simulink library "AssistOn_Gait_Lib"  (R2020a)
settings: Solver=VariableStepAuto  StartTime=0.0  StopTime=10.0  RelTol=1e-3
libraries: xpcethercatlib x12, simulink x3, slrtlib x1
settings Model: Creator=AliYasar  LastModifiedBy=AliYasar

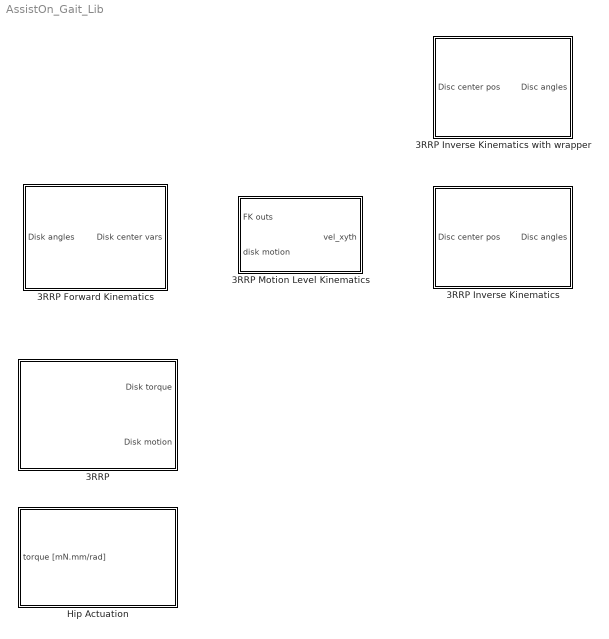
== system AssistOn_Gait_Lib ==
  3RRP : Subsystem  TreatAsAtomicUnit=on
  3RRP Forward Kinematics : Subsystem
      settings: MinAlgLoopOccurrences=on
  3RRP Inverse Kinematics : Subsystem
      settings: MinAlgLoopOccurrences=on
  3RRP Inverse Kinematics with wrapper : Subsystem
      settings: MinAlgLoopOccurrences=on
  3RRP Motion Level Kinematics : Subsystem
  Hip Actuation : Subsystem

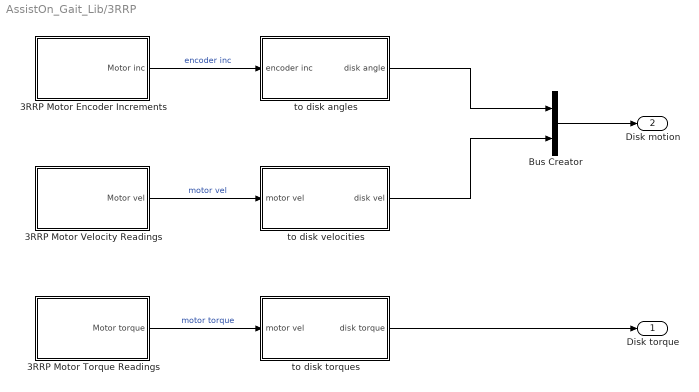
== system AssistOn_Gait_Lib/3RRP ==
  3RRP Motor Encoder Increments : Subsystem
  3RRP Motor Torque Readings : Subsystem
  3RRP Motor Velocity Readings : Subsystem
  Bus Creator : BusCreator  Inputs=2
  to disk angles : Subsystem
  to disk torques : Subsystem
  to disk velocities : Subsystem
  Disk torque : Outport  VectorParamsAs1DForOutWhenUnconnected=off
  Disk motion : Outport  Port=2  VectorParamsAs1DForOutWhenUnconnected=off
  wires:
  Bus Creator/1 -> Disk motion/1
  3RRP Motor Velocity Readings/1(Motor vel) -> to disk velocities/1(motor vel)  "motor vel"
  3RRP Motor Encoder Increments/1(Motor inc) -> to disk angles/1(encoder inc)  "encoder inc"
  to disk angles/1(disk angle) -> Bus Creator/1
  to disk velocities/1(disk vel) -> Bus Creator/2
  3RRP Motor Torque Readings/1(Motor torque) -> to disk torques/1(motor vel)  "motor torque"
  to disk torques/1(disk torque) -> Disk torque/1

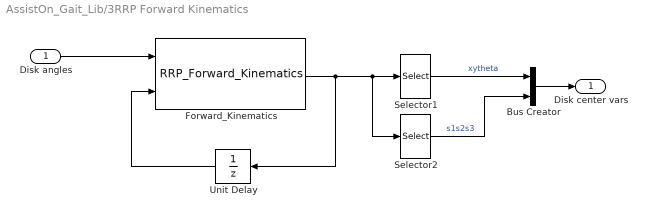
== system AssistOn_Gait_Lib/3RRP Forward Kinematics ==
  Disk angles : Inport
  Bus Creator : BusCreator  Inputs=2
  Forward_Kinematics : S-Function  FunctionName=RRP_Forward_Kinematics  SFunctionModules=RRP_Forward_Kinematics_wrapper  SFunctionDeploymentMode=off  EnableBusSupport=off
  Selector1 : Selector  InputPortWidth=6  IndexOptions=Index vector (dialog)  Indices=[1 2 3]  OutputSizes=1
  Selector2 : Selector  InputPortWidth=6  IndexOptions=Index vector (dialog)  Indices=[4 5 6]  OutputSizes=1
  Unit Delay : UnitDelay  InitialCondition=[0 0 0 151.28 151.28 151.28]  SampleTime=-1  HasFrameUpgradeWarning=on
  Disk center vars : Outport  VectorParamsAs1DForOutWhenUnconnected=off
  wires:
  Unit Delay/1 -> Forward_Kinematics/2
  Forward_Kinematics/1 -> Unit Delay/1, Selector2/1, Selector1/1
  Disk angles/1 -> Forward_Kinematics/1
  Bus Creator/1 -> Disk center vars/1
  Selector1/1 -> Bus Creator/1  "xytheta"
  Selector2/1 -> Bus Creator/2  "s1s2s3"

== system AssistOn_Gait_Lib/3RRP Inverse Kinematics ==
  Disc center pos : Inport
  S-Function : S-Function  FunctionName=RRP_Inverse_Kinematics  SFunctionModules='RRP_Inverse_Kinematics_wrapper'  SFunctionDeploymentMode=off  EnableBusSupport=off
  Unit Delay : UnitDelay  InitialCondition=[2*pi/3,-2*pi/3,0,151.28,151.28,151.28]  SampleTime=-1  HasFrameUpgradeWarning=on
  no op : Subsystem
  Disc angles : Outport
  wires:
  Disc center pos/1 -> S-Function/1
  Unit Delay/1 -> S-Function/2
  S-Function/1 -> no op/1(IK solution)
  no op/1(Pos) -> Disc angles/1
  no op/2(Corrected IK solution) -> Unit Delay/1

== system AssistOn_Gait_Lib/3RRP Inverse Kinematics with wrapper ==
  Disc center pos : Inport
  S-Function : S-Function  FunctionName=RRP_Inverse_Kinematics  SFunctionModules='RRP_Inverse_Kinematics_wrapper'  SFunctionDeploymentMode=off  EnableBusSupport=off
  Unit Delay : UnitDelay  InitialCondition=[2*pi/3,-2*pi/3,0,151.28,151.28,151.28]  SampleTime=-1  HasFrameUpgradeWarning=on
  "wrap position to [-pi, pi]" : Subsystem
  Disc angles : Outport
  wires:
  "wrap position to [-pi, pi]"/2(Corrected IK solution) -> Unit Delay/1
  "wrap position to [-pi, pi]"/1(Pos) -> Disc angles/1
  S-Function/1 -> "wrap position to [-pi, pi]"/1(IK solution)
  Unit Delay/1 -> S-Function/2
  Disc center pos/1 -> S-Function/1

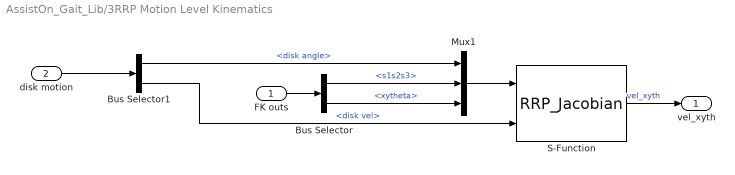
== system AssistOn_Gait_Lib/3RRP Motion Level Kinematics ==
  FK outs : Inport
  disk motion : Inport  Port=2
  Bus Selector : BusSelector  OutputSignals=s1s2s3,xytheta
  Bus Selector1 : BusSelector  OutputSignals=disk angle,disk vel
  Mux1 : Mux  Inputs=3
  S-Function : S-Function  FunctionName=RRP_Jacobian  SFunctionModules='RRP_Jacobian_wrapper'  SFunctionDeploymentMode=off  EnableBusSupport=off
  vel_xyth : Outport
  wires:
  Mux1/1 -> S-Function/1
  FK outs/1 -> Bus Selector/1
  S-Function/1 -> vel_xyth/1  "vel_xyth"
  disk motion/1 -> Bus Selector1/1
  Bus Selector/1 -> Mux1/2  "<s1s2s3>"
  Bus Selector/2 -> Mux1/3  "<xytheta>"
  Bus Selector1/1 -> Mux1/1  "<disk angle>"
  Bus Selector1/2 -> S-Function/2  "<disk vel>"

== system AssistOn_Gait_Lib/Hip Actuation ==
  torque [mN.mm/rad] : Inport
  M1 Target Torque : xpcethercatlib/EtherCAT PDO Transmit   Priority=3  sig_name=Drive 1 (MAXPOS).Module 1 (CST Mode).CST Outputs.Target Torque  sig_offset=656  sig_type=int16  type_size=16  sig_dim=1  device_id=0  sample_time=0.001000
      settings: SourceProductBaseCode=XP
  M2 Target Torque : xpcethercatlib/EtherCAT PDO Transmit   Priority=3  sig_name=Drive 2 (MAXPOS).Module 1 (CST Mode).CST Outputs.TargetTorque  sig_offset=768  sig_type=int16  type_size=16  sig_dim=1  device_id=0  sample_time=0.001000
      settings: SourceProductBaseCode=XP
  M3 Target Torque : xpcethercatlib/EtherCAT PDO Transmit   Priority=3  sig_name=Drive 3 (MAXPOS).Module 1 (CST Mode).CST Outputs.TargetTorque  sig_offset=880  sig_type=int16  type_size=16  sig_dim=1  device_id=0  sample_time=0.001000
      settings: SourceProductBaseCode=XP
  Target Torque : Subsystem
  wires:
  torque [mN.mm/rad]/1 -> Target Torque/1(torque)
  Target Torque/1(M1_torque) -> M1 Target Torque/1
  Target Torque/2(M2_torque) -> M2 Target Torque/1
  Target Torque/3(M3_torque) -> M3 Target Torque/1

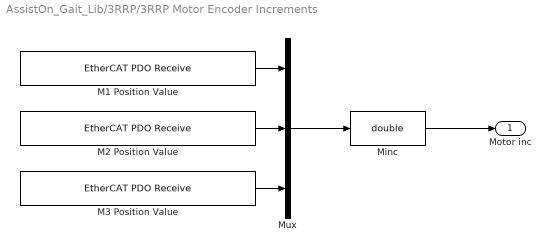
== system AssistOn_Gait_Lib/3RRP/3RRP Motor Encoder Increments ==
  M1 Position Value : xpcethercatlib/EtherCAT PDO Receive  Priority=2  sig_name=Drive 1 (MAXPOS).Module 1 (CST Mode).CST Inputs.PositionActualValue  sig_offset=568  sig_type=int32  type_size=32  sig_dim=1  device_id=0  sample_time=0.001000
      settings: SourceProductBaseCode=XP
  M2 Position Value : xpcethercatlib/EtherCAT PDO Receive  Priority=2  sig_name=Drive 2 (MAXPOS).Module 1 (CST Mode).CST Inputs.PositionActualValue  sig_offset=680  sig_type=int32  type_size=32  sig_dim=1  device_id=0  sample_time=0.001000
      settings: SourceProductBaseCode=XP
  M3 Position Value : xpcethercatlib/EtherCAT PDO Receive  Priority=2  sig_name=Drive 3 (MAXPOS).Module 1 (CST Mode).CST Inputs.PositionActualValue  sig_offset=792  sig_type=int32  type_size=32  sig_dim=1  device_id=0  sample_time=0.001000
      settings: SourceProductBaseCode=XP
  Minc : DataTypeConversion  OutDataTypeStr=double
  Mux : Mux  Inputs=3
  Motor inc : Outport  VectorParamsAs1DForOutWhenUnconnected=off
  wires:
  Minc/1 -> Motor inc/1
  M3 Position Value/1 -> Mux/3
  M1 Position Value/1 -> Mux/1
  M2 Position Value/1 -> Mux/2
  Mux/1 -> Minc/1

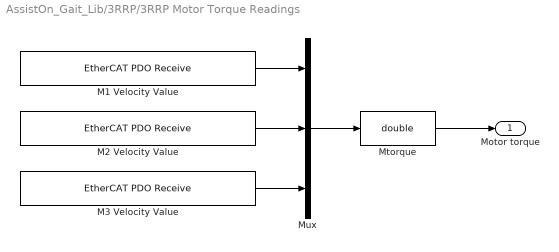
== system AssistOn_Gait_Lib/3RRP/3RRP Motor Torque Readings ==
  M1 Velocity Value : xpcethercatlib/EtherCAT PDO Receive  Priority=2  sig_name=Drive 1 (MAXPOS).Module 1 (CST Mode).CST Inputs.Velocity Actual Value Averaged  sig_offset=632  sig_type=int32  type_size=32  sig_dim=1  device_id=0  sample_time=0.001000
      settings: SourceProductBaseCode=XP
  M2 Velocity Value : xpcethercatlib/EtherCAT PDO Receive  Priority=2  sig_name=Drive 2 (MAXPOS).Module 1 (CST Mode).CST Inputs.Velocity Actual Value Averaged  sig_offset=744  sig_type=int32  type_size=32  sig_dim=1  device_id=0  sample_time=0.001000
      settings: SourceProductBaseCode=XP
  M3 Velocity Value : xpcethercatlib/EtherCAT PDO Receive  Priority=2  sig_name=Drive 3 (MAXPOS).Module 1 (CST Mode).CST Inputs.Velocity Actual Value Averaged  sig_offset=872  sig_type=int32  type_size=32  sig_dim=1  device_id=0  sample_time=0.001000
      settings: SourceProductBaseCode=XP
  Mtorque : DataTypeConversion  OutDataTypeStr=double
  Mux : Mux  Inputs=3
  Motor torque : Outport
  wires:
  Mtorque/1 -> Motor torque/1
  Mux/1 -> Mtorque/1
  M3 Velocity Value/1 -> Mux/3
  M2 Velocity Value/1 -> Mux/2
  M1 Velocity Value/1 -> Mux/1

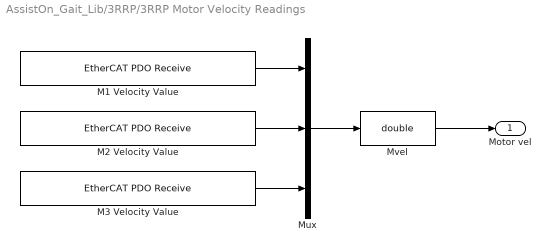
== system AssistOn_Gait_Lib/3RRP/3RRP Motor Velocity Readings ==
  M1 Velocity Value : xpcethercatlib/EtherCAT PDO Receive  Priority=2  sig_name=Drive 1 (MAXPOS).Module 1 (CST Mode).CST Inputs.Velocity Actual Value Averaged  sig_offset=632  sig_type=int32  type_size=32  sig_dim=1  device_id=0  sample_time=0.001000
      settings: SourceProductBaseCode=XP
  M2 Velocity Value : xpcethercatlib/EtherCAT PDO Receive  Priority=2  sig_name=Drive 2 (MAXPOS).Module 1 (CST Mode).CST Inputs.Velocity Actual Value Averaged  sig_offset=744  sig_type=int32  type_size=32  sig_dim=1  device_id=0  sample_time=0.001000
      settings: SourceProductBaseCode=XP
  M3 Velocity Value : xpcethercatlib/EtherCAT PDO Receive  Priority=2  sig_name=Drive 3 (MAXPOS).Module 1 (CST Mode).CST Inputs.Velocity Actual Value Averaged  sig_offset=872  sig_type=int32  type_size=32  sig_dim=1  device_id=0  sample_time=0.001000
      settings: SourceProductBaseCode=XP
  Mux : Mux  Inputs=3
  Mvel : DataTypeConversion  OutDataTypeStr=double
  Motor vel : Outport
  wires:
  M1 Velocity Value/1 -> Mux/1
  M2 Velocity Value/1 -> Mux/2
  M3 Velocity Value/1 -> Mux/3
  Mux/1 -> Mvel/1
  Mvel/1 -> Motor vel/1

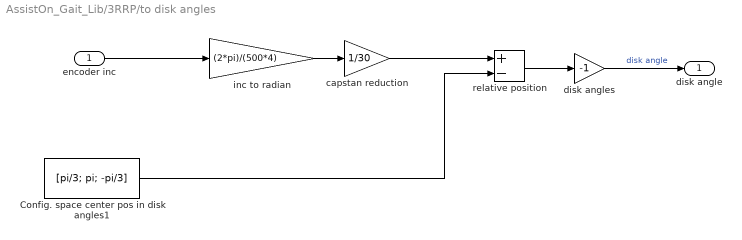
== system AssistOn_Gait_Lib/3RRP/to disk angles ==
  encoder inc : Inport
  Config. space center pos in disk angles1 : Constant  Value=[pi/3; pi; -pi/3]
  capstan reduction : Gain  Gain=1/30
  disk angles : Gain  Gain=-1
  inc to radian : Gain  Gain=(2*pi)/(500*4)
  relative position : Sum  Inputs=+-
  disk angle : Outport
  wires:
  inc to radian/1 -> capstan reduction/1
  capstan reduction/1 -> relative position/1
  encoder inc/1 -> inc to radian/1
  Config. space center pos in disk angles1/1 -> relative position/2
  relative position/1 -> disk angles/1
  disk angles/1 -> disk angle/1  "disk angle"

== system AssistOn_Gait_Lib/3RRP/to disk torques ==
  motor vel : Inport
  capstan reduction : Gain  Gain=30
  disk torques : Gain  Gain=-1
  torque mapping : Gain  Gain=123/1000  OutDataTypeStr=double
  disk torque : Outport
  wires:
  disk torques/1 -> disk torque/1  "disk torque"
  torque mapping/1 -> capstan reduction/1
  motor vel/1 -> torque mapping/1
  capstan reduction/1 -> disk torques/1

== system AssistOn_Gait_Lib/3RRP/to disk velocities ==
  motor vel : Inport
  capstan reduction : Gain  Gain=1/30
  disk vels : Gain  Gain=-1
  rpm to rad/s : Gain  Gain=(2*pi)/60
  disk vel : Outport
  wires:
  capstan reduction/1 -> disk vels/1
  motor vel/1 -> rpm to rad/s/1
  rpm to rad/s/1 -> capstan reduction/1
  disk vels/1 -> disk vel/1  "disk vel"

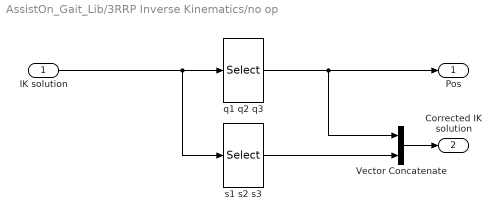
== system AssistOn_Gait_Lib/3RRP Inverse Kinematics/no op ==
  IK solution : Inport
  Vector Concatenate : Concatenate
  q1 q2 q3 : Selector  IndexMode=Zero-based  InputPortWidth=6  IndexOptions=Index vector (dialog)  Indices=[0 1 2]  OutputSizes=1
  s1 s2 s3 : Selector  IndexMode=Zero-based  InputPortWidth=6  IndexOptions=Index vector (dialog)  Indices=[3 4 5]  OutputSizes=1
  Pos : Outport
  Corrected IK solution : Outport  Port=2
  wires:
  IK solution/1 -> s1 s2 s3/1, q1 q2 q3/1
  s1 s2 s3/1 -> Vector Concatenate/2
  Vector Concatenate/1 -> Corrected IK solution/1
  q1 q2 q3/1 -> Vector Concatenate/1, Pos/1

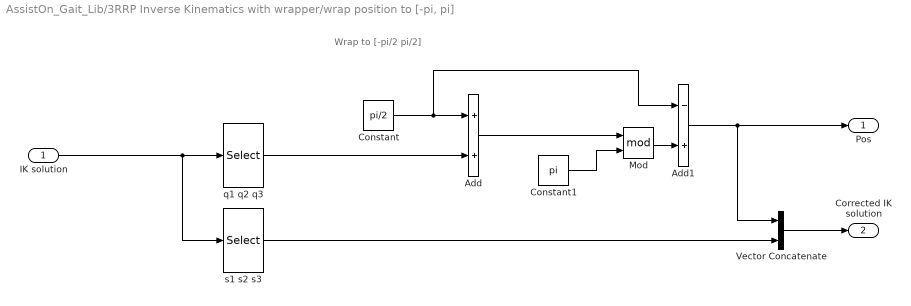
== system AssistOn_Gait_Lib/3RRP Inverse Kinematics with wrapper/wrap position to [-pi, pi] ==
  note: Wrap to [-pi/2 pi/2]
  IK solution : Inport
  Add : Sum
  Add1 : Sum  Inputs=-+
  Constant : Constant  Value=pi/2
  Constant1 : Constant  Value=pi
  Mod : Math  Operator=mod  SaturateOnIntegerOverflow=on
  Vector Concatenate : Concatenate
  q1 q2 q3 : Selector  IndexMode=Zero-based  InputPortWidth=6  IndexOptions=Index vector (dialog)  Indices=[0 1 2]  OutputSizes=1
  s1 s2 s3 : Selector  IndexMode=Zero-based  InputPortWidth=6  IndexOptions=Index vector (dialog)  Indices=[3 4 5]  OutputSizes=1
  Pos : Outport
  Corrected IK solution : Outport  Port=2
  wires:
  Vector Concatenate/1 -> Corrected IK solution/1
  Add1/1 -> Pos/1, Vector Concatenate/1
  Add/1 -> Mod/1
  Constant/1 -> Add/1, Add1/1
  q1 q2 q3/1 -> Add/2
  s1 s2 s3/1 -> Vector Concatenate/2
  Mod/1 -> Add1/2
  IK solution/1 -> q1 q2 q3/1, s1 s2 s3/1
  Constant1/1 -> Mod/2

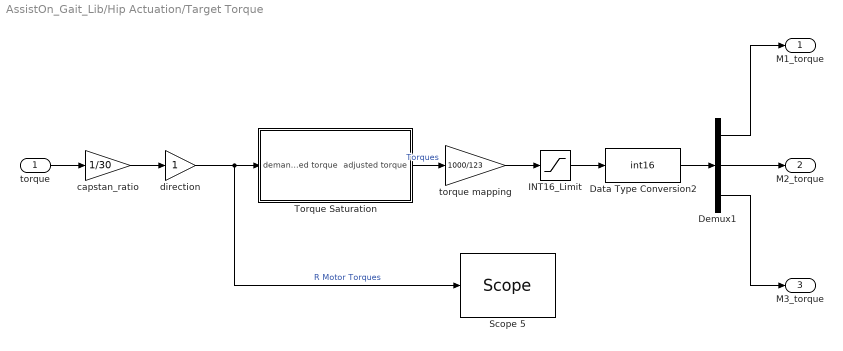
== system AssistOn_Gait_Lib/Hip Actuation/Target Torque ==
  torque : Inport
  Data Type Conversion2 : DataTypeConversion  OutDataTypeStr=int16
  Demux1 : Demux  Outputs=3
  INT16_Limit : Saturate  UpperLimit=[2^15-1 2^15-1 2^15-1]  LowerLimit=[-2^15 -2^15 -2^15]
  Scope 5 : slrtlib/Displays and Logging/Scope   scopeno=1  scopetype=Target  autostart=on  viewmode=Numerical  formatstr='%15.6f'  grid=on  ylimits=pi/6*[-1, 1]  nosamples=5  noprepostsamples=0  interleave=10  triggermode=FreeRun  triggersignal=1  trigsignalfromport=off  triggerlevel=0.0  triggerslope=Either  triggerscope=1  triggersample=0  filename=rhipinc.dat  mode=Lazy  writesize=512  autorestart=off  dynamicfilemode=off  maxwritefilesize=512*1024^2
  Torque Saturation : Subsystem
  capstan_ratio : Gain  Gain=1/30
  direction : Gain  OutDataTypeStr=double
  torque mapping : Gain  Gain=1000/123  OutDataTypeStr=double
  M1_torque : Outport  VectorParamsAs1DForOutWhenUnconnected=off
  M2_torque : Outport  Port=2  VectorParamsAs1DForOutWhenUnconnected=off
  M3_torque : Outport  Port=3  VectorParamsAs1DForOutWhenUnconnected=off
  wires:
  direction/1 -> Scope 5/1, Torque Saturation/1(demanded torque)  "R Motor Torques"
  torque/1 -> capstan_ratio/1
  capstan_ratio/1 -> direction/1
  Data Type Conversion2/1 -> Demux1/1
  INT16_Limit/1 -> Data Type Conversion2/1
  torque mapping/1 -> INT16_Limit/1
  Demux1/1 -> M1_torque/1
  Demux1/2 -> M2_torque/1
  Demux1/3 -> M3_torque/1
  Torque Saturation/1(adjusted torque) -> torque mapping/1  "Torques"

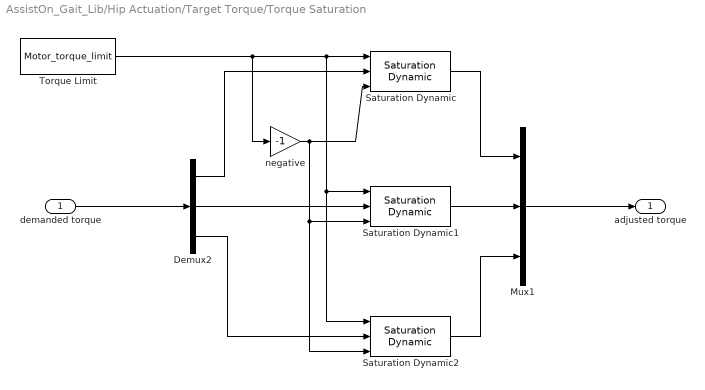
== system AssistOn_Gait_Lib/Hip Actuation/Target Torque/Torque Saturation ==
  demanded torque : Inport
  Demux2 : Demux  Outputs=3
  Mux1 : Mux  Inputs=3
  Saturation Dynamic : simulink/Discontinuities/Saturation Dynamic  OutMin=[]  OutMax=[]  OutDataTypeStr=Inherit: Same as second input  OutDataType=fixdt(1, 16)  OutScaling=2^-10  RndMeth=Simplest  DoSatur=off
  Saturation Dynamic1 : simulink/Discontinuities/Saturation Dynamic  OutMin=[]  OutMax=[]  OutDataTypeStr=Inherit: Same as second input  OutDataType=fixdt(1, 16)  OutScaling=2^-10  RndMeth=Simplest  DoSatur=off
  Saturation Dynamic2 : simulink/Discontinuities/Saturation Dynamic  OutMin=[]  OutMax=[]  OutDataTypeStr=Inherit: Same as second input  OutDataType=fixdt(1, 16)  OutScaling=2^-10  RndMeth=Simplest  DoSatur=off
  Torque Limit : DataStoreRead  DataStoreName=Motor_torque_limit
  negative : Gain  Gain=-1  OutDataTypeStr=double
  adjusted torque : Outport
  wires:
  Torque Limit/1 -> Saturation Dynamic/1, Saturation Dynamic1/1, Saturation Dynamic2/1, negative/1
  Demux2/2 -> Saturation Dynamic1/2
  Demux2/1 -> Saturation Dynamic/2
  Mux1/1 -> adjusted torque/1
  Saturation Dynamic2/1 -> Mux1/3
  negative/1 -> Saturation Dynamic/3, Saturation Dynamic2/3, Saturation Dynamic1/3
  Saturation Dynamic1/1 -> Mux1/2
  Saturation Dynamic/1 -> Mux1/1
  Demux2/3 -> Saturation Dynamic2/2
  demanded torque/1 -> Demux2/1
